simulink model "Animation_square_v15"  (R2022b)
settings: Solver=VariableStepAuto  StartTime=0.0  StopTime=30  RelTol=1e-3
model workspace (MAT data in the model file):
  rotation_orig = [0 0 0]
libraries: sim3dcameralib x2, uavsim3dlib x2, dspvision x2, simulink x1, sim3dlib x1, visionsinks x1
settings Model: Creator=David  LastModifiedBy=David
settings DebuggingCC: UnconnectedInputMsg=warning  UnconnectedOutputMsg=warning  UnconnectedLineMsg=warning
settings ModelReferenceCC: EnableRefExpFcnMdlSchedulingChecks=on
settings RTWCC: DLArmComputeVersion=19.05

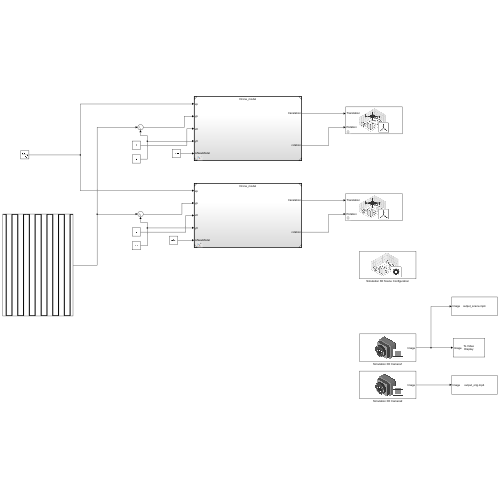
[thumbnail: Simulink's stored preview of the top-level diagram]
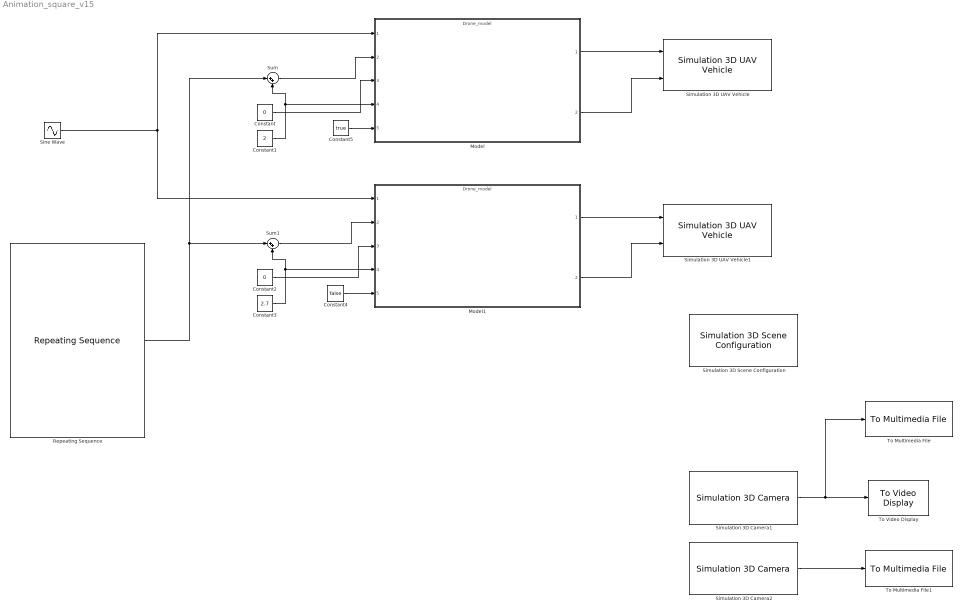
== system Animation_square_v15 ==
  Constant : Constant  Value=0
  Constant1 : Constant  Value=2
  Constant2 : Constant  Value=0
  Constant3 : Constant  Value=2.7
  Constant4 : Constant  Value=false
  Constant5 : Constant  Value=true
  Model : ModelReference  ModelNameDialog=Drone_model.slx  SimulationMode=Normal  ModelReferenceVersion=1.17
  Model1 : ModelReference  ModelNameDialog=Drone_model.slx  SimulationMode=Normal  ModelReferenceVersion=1.17
  Repeating Sequence : simulink/Sources/Repeating Sequence  rep_seq_t=[0, 2*pi/6-10^(-6),2*pi/6,2*3*pi/6-10^(-6),2*3*pi/6,2*5*pi/6-10^(-6),2*5*pi/6,2*7*pi/6-10^(-6),2*7*pi/6,2*8*pi/6]  rep_seq_y=[0,0,-1,-1,0,0,-1,-1,0,0]
  Simulation 3D Camera1 : sim3dcameralib/Simulation 3D Camera  Priority=1  sensorTag=Sim3dSensor2  sensorId=2  sensorName=Sim3dSensor2  vehTagList={'Scene Origin';'SimulinkVehicle1';'SimulinkVehicle2'}  vehTag=Scene Origin  mountLoc=Origin  offsetFlag=on  tmountOffset=[-3.3, 1.425, 2]  extTmount=off  rmountOffset=[0, 0, 0]  extRmount=off  FocalLength=[1109, 1109]  OpticalCenter=[960, 540]  ImageSize=[1080, 1920]  RadialDistortion=[0, 0]  TangentialDistortion=[0, 0]  SensorSkew=0  DepthOutportEnabled=off  SemanticOutportEnabled=off  TransformOutportEnabled=off  SampleTime=-1  mountPoint=[-3.3 -1.425 2]  mountOrientation=[0 0 0]  aMode=4  ID=2
  Simulation 3D Camera2 : sim3dcameralib/Simulation 3D Camera  Priority=1  sensorTag=Sim3dSensor3  sensorId=3  sensorName=Sim3dSensor3  vehTagList={'Scene Origin';'SimulinkVehicle1';'SimulinkVehicle2'}  vehTag=SimulinkVehicle2  mountLoc=Origin  offsetFlag=on  tmountOffset=[-1.5, 0, 0]  extTmount=off  rmountOffset=[0,0,0]  extRmount=off  FocalLength=[1109, 1109]  OpticalCenter=[960, 540]  ImageSize=[1080, 1920]  RadialDistortion=[0, 0]  TangentialDistortion=[0, 0]  SensorSkew=0  DepthOutportEnabled=off  SemanticOutportEnabled=off  TransformOutportEnabled=off  SampleTime=-1  mountPoint=[-1.5 0 0]  mountOrientation=[0 0 0]  aMode=4  ID=3
  Simulation 3D Scene Configuration : sim3dlib/Simulation 3D Scene Configuration  Priority=0  ProjectFormat=Default Scenes  SceneDesc=US city block  ProjectName=C:\Program Files\MATLAB\R2022b\toolbox\shared\sim3d_projects\automotive_project\UE4\WindowsNoEditor\VehicleSimulation.exe  ScenePath=/Game/Maps/USCityBlock  EnableOpenDRIVE=off  vehTagList={'Scene Origin';'SimulinkVehicle1';'SimulinkVehicle2'}  vehTag=Scene Origin  OpVisEn=off  Ts=1/60  EnableWindow=off  EnableRemoteAccess=off  EnableWeather=off  SunAltitude=40.0  SunAzimuth=90  clouds=10  wind=1  fog=0  rain=0  EnableGeospatial=off  OriginHeight=200  OriginLatitude=40.744652  OriginLongitude=-73.988864  MapStyle=Aerial  AdditionalAssetIDs=[]  UseAdvancedSunSky=off  SolarTime=11  TimeZone=-5  Day=21  Month=9  Year=2022  UseDaylightSavingTime=on  DSTStartDay=10  DSTStartMonth=3  DSTEndDay=3  DSTEndMonth=11  DSTSwitchHour=2  sensorTag=MainCamera1  sensorId=1  sensorName=MainCamera1  mountLoc=Origin  offsetFlag=off  tmountOffset=[0, 0, 0]  rmountOffset=[0, 0, 0]  HorizontalResolution=1280  VerticalResolution=720  HorizontalFOV=60  mountPoint=[0 0 0]  mountOrientation=[0 0 0]  aMode=4  ID=1  GeoTrigger=Inactive
  Simulation 3D UAV Vehicle : uavsim3dlib/Simulation 3D UAV Vehicle  Priority=-1  Mesh=Quadrotor  MeshPath=/MathWorksUAVContent/UAVs/HexaRotorUAV/HexaRotor.HexaRotor  Color=Black  ActorName=SimulinkVehicle1  InitialTranslation=[0 0 2]  InitialRotation=[0 0 0]  SampleTime=-1  ActorType=SimulinkVehicle  ID=1  aMode=4  ActorTag=SimulinkVehicle1
  Simulation 3D UAV Vehicle1 : uavsim3dlib/Simulation 3D UAV Vehicle  Priority=-1  Mesh=Quadrotor  MeshPath=/MathWorksUAVContent/UAVs/HexaRotorUAV/HexaRotor.HexaRotor  Color=Blue  ActorName=SimulinkVehicle2  InitialTranslation=[0 0 2.5]  InitialRotation=[0 0 0]  SampleTime=-1  ActorType=SimulinkVehicle  ID=2  aMode=4  ActorTag=SimulinkVehicle2
  Sine Wave : Sin  Frequency=1.5  SampleTime=0
  Sum : Sum  Inputs=|++
  Sum1 : Sum  Inputs=|++
  To Multimedia File : dspvision/To Multimedia File  outputFilename=output_scene.mp4  streamSelection=Video only  videoCompressor=None (uncompressed)  audioCompressor=None (uncompressed)  imagePorts=One multidimensional signal  fileType=MPEG4  audioDatatype=Determine from input data type  fourcc=RGB  videoQuality=75  mj2000CompFactor=10
  To Multimedia File1 : dspvision/To Multimedia File  outputFilename=output_orig.mp4  streamSelection=Video only  videoCompressor=None (uncompressed)  audioCompressor=None (uncompressed)  imagePorts=One multidimensional signal  fileType=MPEG4  audioDatatype=Determine from input data type  fourcc=RGB  videoQuality=75  mj2000CompFactor=10
  To Video Display : visionsinks/To Video Display  Priority=2  windowSizeMode=Normal  openAtMdlStart=on  fullScreen=off  videoWindowX=536805376  videoWindowY=536805376  saveWindowSize=off  videoWindowWidth=1920  videoWindowHeight=1061  inputColorFormat=RGB  inputType=Obsolete  imagePorts=One multidimensional signal  OutputDevice=On-screen video monitor  dataOrg=Column-major  isWindowOpen=off
  wires:
  Simulation 3D Camera1/1 -> To Video Display/1, To Multimedia File/1
  Model/2 -> Simulation 3D UAV Vehicle/2
  Sum/1 -> Model/2
  Constant/1 -> Model/3
  Constant1/1 -> Sum/2, Model/4
  Model/1 -> Simulation 3D UAV Vehicle/1
  Model1/1 -> Simulation 3D UAV Vehicle1/1
  Constant3/1 -> Sum1/2, Model1/4
  Model1/2 -> Simulation 3D UAV Vehicle1/2
  Sum1/1 -> Model1/2
  Constant2/1 -> Model1/3
  Simulation 3D Camera2/1 -> To Multimedia File1/1
  Sine Wave/1 -> Model1/1, Model/1
  Repeating Sequence/1 -> Sum1/1, Sum/1
  Constant4/1 -> Model1/5
  Constant5/1 -> Model/5
